simulink model "Modelo_del_sistema"  (R2018a)
settings: Solver=VariableStepAuto  StartTime=0  StopTime=2678400  FixedStep=45  RelTol=1e-3  EnableMultiTasking=on
libraries: simulink x2
(part 2 of 2)

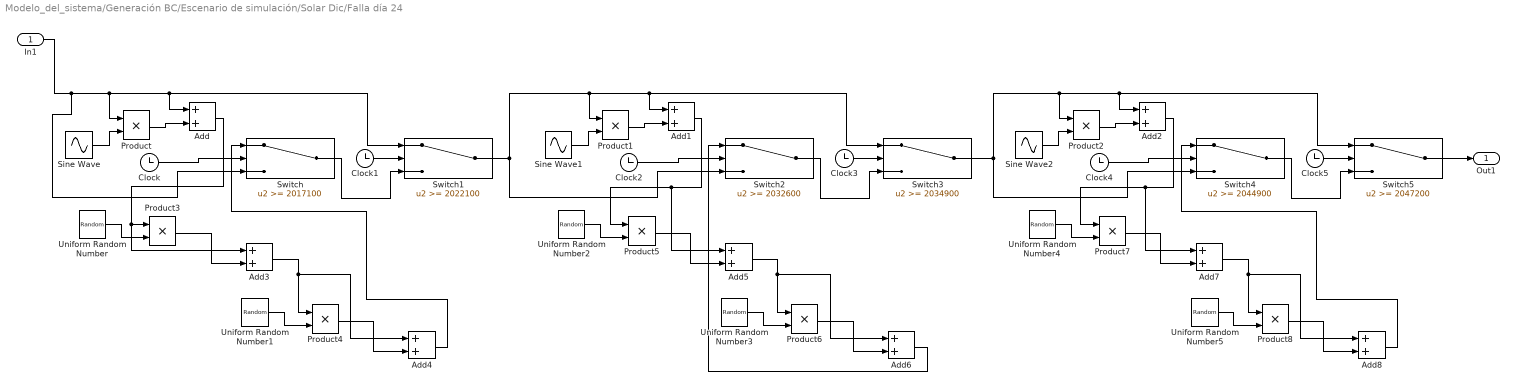
== system Modelo_del_sistema/Generación BC/Escenario de simulación/Solar Dic/Falla día 24 ==
  In1 : Inport
  Add{,1..8} (9 alike) : Sum
  Clock{,1..5} (6 alike) : Clock
  Product{,1..8} (9 alike) : Product
  Sine Wave : Sin  Amplitude=0.59  Frequency=0.000628319  Phase=-pi/2+pi/12.5  SampleTime=0
  Sine Wave1 : Sin  Amplitude=0.49  Frequency=0.001365910  Phase=-pi/2-pi/4+pi/92.7  SampleTime=0
  Sine Wave2 : Sin  Amplitude=0.89  Frequency=0.001365910  Phase=-pi/11.5  SampleTime=0
  Switch : Switch  Threshold=2017100
  Switch1 : Switch  Threshold=2022100
  Switch2 : Switch  Threshold=2032600
  Switch3 : Switch  Threshold=2034900
  Switch4 : Switch  Threshold=2044900
  Switch5 : Switch  Threshold=2047200
  Uniform Random Number : UniformRandomNumber  Minimum=-0.5  Maximum=0  Seed=1337  SampleTime=50
  Uniform Random Number1 : UniformRandomNumber  Minimum=-0.25  Maximum=0  Seed=69420  SampleTime=25
  Uniform Random Number2 : UniformRandomNumber  Minimum=-0.5  Maximum=0  Seed=1337  SampleTime=50
  Uniform Random Number3 : UniformRandomNumber  Minimum=-0.25  Maximum=0  Seed=69420  SampleTime=25
  Uniform Random Number4 : UniformRandomNumber  Minimum=-0.5  Maximum=0  Seed=1337  SampleTime=50
  Uniform Random Number5 : UniformRandomNumber  Minimum=-0.25  Maximum=0  Seed=69420  SampleTime=25
  Out1 : Outport
  wires:
  Product/1 -> Add/2
  Clock/1 -> Switch/2
  In1/1 -> Switch/3, Product/1, Add/1, Switch1/1
  Sine Wave/1 -> Product/2
  Clock1/1 -> Switch1/2
  Switch/1 -> Switch1/3
  Product1/1 -> Add1/2
  Clock2/1 -> Switch2/2
  Switch1/1 -> Product1/1, Add1/1, Switch3/1, Switch2/3
  Sine Wave1/1 -> Product1/2
  Clock3/1 -> Switch3/2
  Switch2/1 -> Switch3/3
  Product2/1 -> Add2/2
  Clock4/1 -> Switch4/2
  Switch3/1 -> Product2/1, Add2/1, Switch5/1, Switch4/3
  Sine Wave2/1 -> Product2/2
  Clock5/1 -> Switch5/2
  Switch4/1 -> Switch5/3
  Switch5/1 -> Out1/1
  Add3/1 -> Add4/1, Product4/1
  Product4/1 -> Add4/2
  Add4/1 -> Switch/1
  Uniform Random Number1/1 -> Product4/2
  Add/1 -> Add3/1, Product3/1
  Uniform Random Number/1 -> Product3/2
  Product3/1 -> Add3/2
  Add5/1 -> Add6/1, Product6/1
  Product6/1 -> Add6/2
  Uniform Random Number3/1 -> Product6/2
  Add1/1 -> Add5/1, Product5/1
  Uniform Random Number2/1 -> Product5/2
  Product5/1 -> Add5/2
  Add6/1 -> Switch2/1
  Add7/1 -> Add8/1, Product8/1
  Product8/1 -> Add8/2
  Add8/1 -> Switch4/1
  Uniform Random Number5/1 -> Product8/2
  Add2/1 -> Add7/1, Product7/1
  Uniform Random Number4/1 -> Product7/2
  Product7/1 -> Add7/2

== system Modelo_del_sistema/Generación BC/Escenario de simulación/Solar Dic/Falla día 28 ==
  In1 : Inport
  Add : Sum
  Add1 : Sum
  Add2 : Sum
  Clock : Clock
  Clock1 : Clock
  Product : Product
  Product1 : Product
  Product2 : Product
  Sine Wave : Sin  Amplitude=0.53  Frequency=0.000506708  Phase=pi-pi/4.435  SampleTime=0
  Switch : Switch  Threshold=2357400
  Switch1 : Switch  Threshold=2363600
  Uniform Random Number : UniformRandomNumber  Minimum=-0.5  Maximum=0  Seed=1337  SampleTime=50
  Uniform Random Number1 : UniformRandomNumber  Minimum=-0.25  Maximum=0  Seed=69420  SampleTime=25
  Out1 : Outport
  wires:
  Product/1 -> Add/2
  Clock/1 -> Switch/2
  In1/1 -> Switch/3, Product/1, Add/1, Switch1/1
  Switch1/1 -> Out1/1
  Sine Wave/1 -> Product/2
  Clock1/1 -> Switch1/2
  Switch/1 -> Switch1/3
  Add1/1 -> Add2/1, Product2/1
  Product2/1 -> Add2/2
  Add2/1 -> Switch/1
  Uniform Random Number1/1 -> Product2/2
  Add/1 -> Add1/1, Product1/1
  Uniform Random Number/1 -> Product1/2
  Product1/1 -> Add1/2

== system Modelo_del_sistema/Generación BC/Escenario de simulación/Solar Dic/Falla día 30 ==
  In1 : Inport
  Add : Sum
  Add1 : Sum
  Add2 : Sum
  Clock : Clock
  Clock1 : Clock
  Product : Product
  Product1 : Product
  Product2 : Product
  Sine Wave : Sin  Amplitude=0.84  Frequency=0.000275578  Phase=-pi/2+pi/7.11  SampleTime=0
  Switch : Switch  Threshold=2546300
  Switch1 : Switch  Threshold=2557700
  Uniform Random Number : UniformRandomNumber  Minimum=-0.5  Maximum=0  Seed=1337  SampleTime=50
  Uniform Random Number1 : UniformRandomNumber  Minimum=-0.25  Maximum=0  Seed=69420  SampleTime=25
  Out1 : Outport
  wires:
  Product/1 -> Add/2
  Clock/1 -> Switch/2
  In1/1 -> Switch/3, Product/1, Add/1, Switch1/1
  Switch1/1 -> Out1/1
  Sine Wave/1 -> Product/2
  Clock1/1 -> Switch1/2
  Switch/1 -> Switch1/3
  Add1/1 -> Add2/1, Product2/1
  Product2/1 -> Add2/2
  Add2/1 -> Switch/1
  Uniform Random Number1/1 -> Product2/2
  Add/1 -> Add1/1, Product1/1
  Uniform Random Number/1 -> Product1/2
  Product1/1 -> Add1/2

== system Modelo_del_sistema/Generación BC/Escenario de simulación/Solar Dic/Falla día 4 ==
  In1 : Inport
  Add : Sum
  Add1 : Sum
  Add2 : Sum
  Clock : Clock
  Clock1 : Clock
  Product : Product
  Product1 : Product
  Product2 : Product
  Sine Wave : Sin  Amplitude=0.51  Frequency=1.28228e-4  Phase=pi/2+pi/19.6  SampleTime=0
  Switch : Switch  Threshold=305000
  Switch1 : Switch  Threshold=329500
  Uniform Random Number : UniformRandomNumber  Minimum=-0.5  Maximum=0  Seed=1337  SampleTime=50
  Uniform Random Number1 : UniformRandomNumber  Minimum=-0.25  Maximum=0  Seed=69420  SampleTime=25
  Out1 : Outport
  wires:
  Product/1 -> Add/2
  Clock/1 -> Switch/2
  In1/1 -> Switch/3, Product/1, Add/1, Switch1/1
  Switch1/1 -> Out1/1
  Sine Wave/1 -> Product/2
  Clock1/1 -> Switch1/2
  Switch/1 -> Switch1/3
  Add1/1 -> Add2/1, Product2/1
  Product2/1 -> Add2/2
  Add2/1 -> Switch/1
  Uniform Random Number1/1 -> Product2/2
  Add/1 -> Add1/1, Product1/1
  Uniform Random Number/1 -> Product1/2
  Product1/1 -> Add1/2
